simulink model "Simscape_crane_software_model_use_combined"  (R2016b)
settings: Solver=ode15s  StartTime=0.0  StopTime=30  RelTol=1e-3  EnableMultiTasking=on
values from neighbouring files (symbols this model uses):
  TxBreak = 0    [main.m]    (also in setup.m)
  TxCoulomb = 2.5    [main.m]    (also in setup.m)
  TxVisc = 49.1750    (= 49.175)    [main.m]    (also in setup.m)
  TyBreak = 0    [main.m]    (also in setup.m)
  TyCoulomb = 1.8    [main.m]    (also in setup.m)
  xZero = 0    [main.m]    (also in setup.m)
  yZero = 0    [main.m]    (also in setup.m)
undefined symbols (not defined in the file or in its folder): m, MR, sigbuilder_block, TzBreak, TzCoulomb, X, xRange, Y, yRange, Z, zRange, zZero
undefined symbols (not defined in the file): M, TorqueMultX, TorqueMultY, TorqueMultZ, TxTrans, TyTrans, TyVisc, TzTrans, TzVisc
libraries: sm_lib x146, fl_lib x62, nesl_utility x24, simulink x10, elec_lib x9, sm_double_wishbone_suspension_lib x4, aerolibtransform2 x1
(part 1 of 14)
settings Model: Creator=jsustare  LastModifiedBy=nadeen
settings SolverCC: MaxConsecutiveMinStep=10
settings DataIOCC: SaveFormat=StructureWithTime
settings OptimizationCC: LifeSpan=inf
settings DebuggingCC: AllowSymbolicDim=off  SFUnexpectedBacktrackingDiag=warning  SFNoUnconditionalDefaultTransitionDiag=warning  SFExecutionAtInitializationDiag=none
settings ModelReferenceCC: PropagateSignalLabelsOutOfModel=off
settings GRTTargetCC: TargetLangStandard=C89/C90 (ANSI)
settings ConfigComp: CovMetricSettings=dw  CovHtmlReporting=on  CovSaveCumulativeToWorkspaceVar=on  CovSaveSingleToWorkspaceVar=on  CovExternalEMLEnable=off
settings SimscapeCC: SimscapeLogType=all
settings ConfigurationSet: Description=SimMechanics 2G

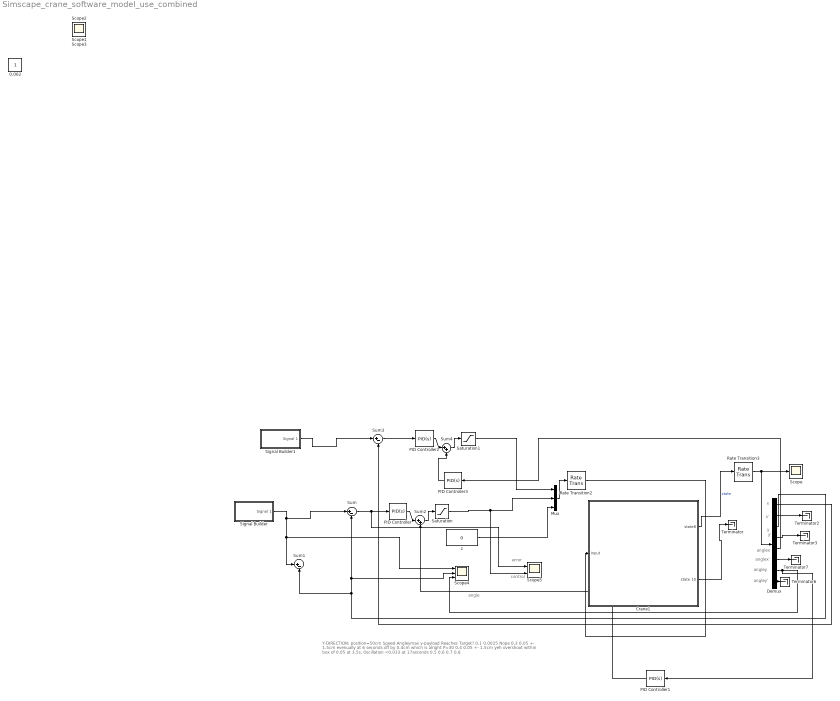
== system Simscape_crane_software_model_use_combined ==
  note: Y-DIRECTION:
      | position=50cm
      | Speed         Angleymax        y-payload       Reaches Target?
      |  0.1               0.0025                                           Nope
      |  0.3                0.05               +- 1.5cm               evenually           at 6 seconds off by 0.4cm which is alright   P=30
      |  0.4                0.05               +- 1.5cm                 yeh                   overshoot within box of 0.05 at 3.5s. Oscillation <0.033 at 17seconds
      |  0.5
      |  0.6
      |  0.7
      |  0.8
  note: control
  note: error
  note: angle
  note: anglex
  note: y'
  note: y
  note: x'
  note: x
  note: anglex'
  note: angley
  note: angley'
  Crane1 : Subsystem  mask{penduMass=m, cartMass=M, MR=MR, xRange=xRange, yRange=yRange, zRange=zRange, xZero=xZero, yZero=yZero, zZero=zZero, TxBreak=TxBreak, TxCoulomb=TxCoulomb, TxVisc=TxVisc, TxTrans=TxTrans, TyBreak=TyBreak, TyCoulomb=TyCoulomb, TyVisc=TyVisc, TyTrans=TyTrans, TzBreak=TzBreak, TzCoulomb=TzCoulomb, TzVisc=TzVisc, TzTrans=TzTrans, Ux=TorqueMultX, Uy=TorqueMultY, Uz=TorqueMultZ}
      mask prompts: penduMass "Pendulum Mass (Kg)"; cartMass "Mass of the cart (Kg)"; MR "Mass of the rail (Kg)"; TxBreak "BreakAwayFriction"; TxCoulomb "Coulomb Friction"; TxVisc "Viscous friction"; TxTrans "Transition coeff"; TyBreak "BreakAwayFriction"; TyCoulomb "Coulomb Friction"; TyVisc "Viscous friction"; TyTrans "Transition coeff"; TzBreak "BreakAwayFriction"; TzCoulomb "Coulomb Friction"; TzVisc "Viscous friction"; TzTrans "Transition coeff"; Ux "Rail motor multiplier (X)"; Uy "Cart motor multiplier (Y)"; Uz "String motor multiplier (Z)"
      mask init:
      | %mass lowSat
      | penduMass=max(penduMass,1e-3);
      | cartMass=max(cartMass,1e-3);
      | MR=max(MR,1e-3);
      | 
      | %zeros saturated
      | xZero=max(xZero,xRange(1));
      | xZero=min(xZero,xRange(2));
      | 
      | yZero=max(yZero,yRange(1));
      | yZero=min(yZero,yRange(2));
      | 
      | zZero=max(zZero,zRange(1));
      | zZero=min(zZero,zRange(2));
      mask DialogControl DescGroupVar Prompt: 3D Crane Simscape model
      mask Display:
